simulink model "foc_hfi"  (R2023a)
settings: Solver=FixedStepAuto  StartTime=0.0  StopTime=1  FixedStep=1e-6  MaxStep=0.00001  RelTol=1e-3
undefined symbols (not defined in the file): DiscIntNeverNeededParam
libraries: slpidlib x4, spsAlphaBetaZerotodq0Lib x1, spsDCVoltageSourceLib x1, spsGroundLib x1, dspfdesign x1, spsPermanentMagnetSynchronousMachineLib x1, simulink x1, spsSVPWMGenerator2LevelLib x1, spsUniversalBridgeLib x1, spsabctoAlphaBetaZeroLib x1, spsdq0toAlphaBetaZeroLib x1, sps_lib x1
settings Model: Creator=28076  LastModifiedBy=28076

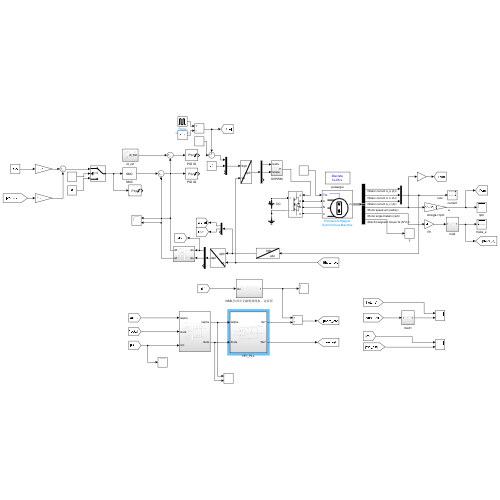
[thumbnail: Simulink's stored preview of the top-level diagram]
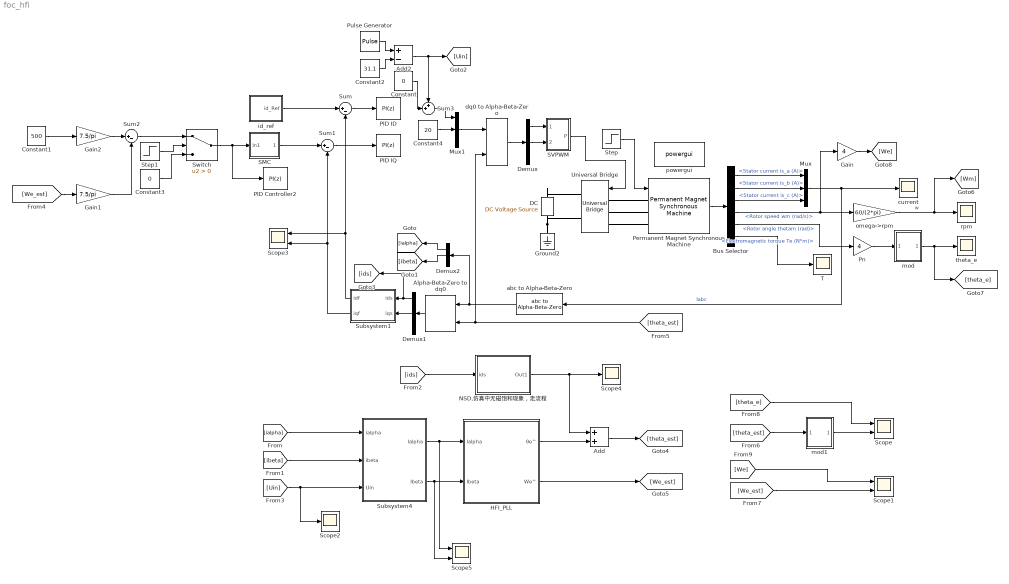
== system foc_hfi ==
  Add : Sum
  Add2 : Sum  Inputs=+-
  Alpha-Beta-Zero to dq0 : spsAlphaBetaZerotodq0Lib/Alpha-Beta-Zero to dq0  Alignment=Aligned with phase A axis
  Bus Selector : BusSelector  OutputSignals=Stator current is_a (A),Stator current is_b (A),Stator current is_c (A),Rotor speed wm (rad/s),Rotor angle thetam (rad),Electromagnetic torque Te (N*m)
  Constant : Constant  Value=0
  Constant1 : Constant  Value=500
  Constant2 : Constant  Value=31.1
  Constant3 : Constant  Value=0
  Constant4 : Constant  Value=20
  "DC " : spsDCVoltageSourceLib/DC Voltage Source  Amplitude=311  Measurements=None
  Demux : Demux  Outputs=3
  Demux1 : Demux  Outputs=3
  Demux2 : Demux  Outputs=3
  Gain : Gain  Gain=4
  Gain1 : Gain  Gain=7.5/pi
  Gain2 : Gain  Gain=7.5/pi
  Ground2 : spsGroundLib/Ground  LConnTagsString=a
  HFI_PLL : Subsystem
  Mux : Mux  Inputs=3
  Mux1 : Mux  Inputs=3
  NSD,仿真中无磁饱和现象，走流程 : Subsystem
  PID Controller2 : slpidlib/PID Controller  Controller=PI  Form=Parallel  TimeDomain=Discrete-time  UseExternalTs=off  SampleTime=1e-4  IntegratorMethod=Forward Euler  FilterMethod=Forward Euler  ControllerParametersSource=internal  P=0.014  I=0.05  UseKiTs=off  D=0  N=100  UseFilter=on  TunerSelectOption=Transfer Function Based (PID Tuner App)  InitialConditionSource=internal  InitialConditionForIntegrator=0  InitialConditionForFilter=0  DifferentiatorICPrevScaledInput=0  ExternalReset=none  TrackingMode=off  Kt=1  LimitOutput=on  SatLimitsSource=internal  UpperSaturationLimit=21  LowerSaturationLimit=-21  LinearizeAsGain=on  AntiWindupMode=none  Kb=1  LimitIntegrator=off  UpperIntegratorSaturationLimit=inf  LowerIntegratorSaturationLimit=-inf  POutMin=[]  POutMax=[]  IOutMin=[]  IOutMax=[]  DOutMin=[]  DOutMax=[]  NOutMin=[]  NOutMax=[]  SumOutMin=[]  SumOutMax=[]  SaturationOutMin=[]  SaturationOutMax=[]  PParamMin=[]  PParamMax=[]  IParamMin=[]  IParamMax=[]  DParamMin=[]  DParamMax=[]  NParamMin=[]  NParamMax=[]  KbParamMin=[]  KbParamMax=[]  KtParamMin=[]  KtParamMax=[]  KbOutMin=[]  KbOutMax=[]  KtOutMin=[]  KtOutMax=[]  IntegratorOutMin=[]  IntegratorOutMax=[]  FilterOutMin=[]  FilterOutMax=[]  SumI1OutMin=[]  SumI1OutMax=[]  SumI2OutMin=[]  SumI2OutMax=[]  SumI3OutMin=[]  SumI3OutMax=[]  SumI4OutMin=[]  SumI4OutMax=[]  SumDOutMin=[]  SumDOutMax=[]  DifferentiatorOutMin=[]  DifferentiatorOutMax=[]  FilterDiffOutCoefMin=[]  FilterDiffOutCoefMax=[]  ReciprocalOutMin=[]  ReciprocalOutMax=[]  SumDenOutMin=[]  SumDenOutMax=[]  SumNumOutMin=[]  SumNumOutMax=[]  DivideOutMin=[]  DivideOutMax=[]  UdiffTsProdOutMin=[]  UdiffTsProdOutMax=[]  NTsProdOutMin=[]  NTsProdOutMax=[]  UintegralTsProdOutMin=[]  UintegralTsProdOutMax=[]  UngainTsProdOutMin=[]  UngainTsProdOutMax=[]  ClampingZeroOutDataTypeStr=Inherit: Inherit via back propagation  ClampingZeroOutMin=[]  ClampingZeroOutMax=[]  FilterDenConstantOutDataTypeStr=Inherit: Inherit via back propagation  FilterDenConstantOutMin=[]  FilterDenConstantOutMax=[]  PCopyOutDataTypeStr=Inherit: Inherit via back propagation  PCopyOutMin=[]  PCopyOutMax=[]  NCopyOutDataTypeStr=Inherit: Inherit via back propagation  NCopyOutMin=[]  NCopyOutMax=[]  IntegratorContinuousStateAttributes=''  IntegratorStateMustResolveToSignalObject=off  IntegratorRTWStateStorageClass=Auto  FilterContinuousStateAttributes=''  FilterStateMustResolveToSignalObject=off  FilterRTWStateStorageClass=Auto  ParallelPVariant=InternalParameters  IdealPVariant=Disabled  IVariant=InternalParameters  DVariant=Disabled  IntegratorVariant=Discrete  SatVariant=Enabled  AWVariant=Passthrough  PCopyVariant=Disabled  TRVariant=Disabled  FdbkBlocksVariant=Forward  IdealPFdbkVariant=Disabled  SatFdbkVariant=Disabled  DerivativeFilterVariant=Disabled  NVariant=Disabled  NCopyVariant=Disabled_SignalSpec  FilterICVariant=Disabled  IntegratorICVariant=InternalICs  ExternalResetVariant=Disabled  TRSumVariant=Passthrough  SumFdbkVariant=Disabled  SumVariant=Sum_PI  TsampFilterVariant=InternalTs  TsampNgainVariant=Passthrough  TsampIntegralVariant=Disabled_SignalSpec  ExternalSaturationOutDataTypeStr=Inherit: Same as second input
  PID ID : slpidlib/PID Controller  Controller=PI  Form=Parallel  TimeDomain=Discrete-time  UseExternalTs=off  SampleTime=1e-4  IntegratorMethod=Forward Euler  FilterMethod=Forward Euler  ControllerParametersSource=internal  P=1100*5.25e-3  I=1100*0.985  UseKiTs=off  D=0  N=100  UseFilter=on  TunerSelectOption=Transfer Function Based (PID Tuner App)  InitialConditionSource=internal  InitialConditionForIntegrator=0  InitialConditionForFilter=0  DifferentiatorICPrevScaledInput=0  ExternalReset=none  TrackingMode=off  Kt=1  LimitOutput=on  SatLimitsSource=internal  UpperSaturationLimit=311/sqrt(3)  LowerSaturationLimit=-311/sqrt(3)  LinearizeAsGain=on  AntiWindupMode=none  Kb=1  LimitIntegrator=off  UpperIntegratorSaturationLimit=inf  LowerIntegratorSaturationLimit=-inf  POutMin=[]  POutMax=[]  IOutMin=[]  IOutMax=[]  DOutMin=[]  DOutMax=[]  NOutMin=[]  NOutMax=[]  SumOutMin=[]  SumOutMax=[]  SaturationOutMin=[]  SaturationOutMax=[]  PParamMin=[]  PParamMax=[]  IParamMin=[]  IParamMax=[]  DParamMin=[]  DParamMax=[]  NParamMin=[]  NParamMax=[]  KbParamMin=[]  KbParamMax=[]  KtParamMin=[]  KtParamMax=[]  KbOutMin=[]  KbOutMax=[]  KtOutMin=[]  KtOutMax=[]  IntegratorOutMin=[]  IntegratorOutMax=[]  FilterOutMin=[]  FilterOutMax=[]  SumI1OutMin=[]  SumI1OutMax=[]  SumI2OutMin=[]  SumI2OutMax=[]  SumI3OutMin=[]  SumI3OutMax=[]  SumI4OutMin=[]  SumI4OutMax=[]  SumDOutMin=[]  SumDOutMax=[]  DifferentiatorOutMin=[]  DifferentiatorOutMax=[]  FilterDiffOutCoefMin=[]  FilterDiffOutCoefMax=[]  ReciprocalOutMin=[]  ReciprocalOutMax=[]  SumDenOutMin=[]  SumDenOutMax=[]  SumNumOutMin=[]  SumNumOutMax=[]  DivideOutMin=[]  DivideOutMax=[]  UdiffTsProdOutMin=[]  UdiffTsProdOutMax=[]  NTsProdOutMin=[]  NTsProdOutMax=[]  UintegralTsProdOutMin=[]  UintegralTsProdOutMax=[]  UngainTsProdOutMin=[]  UngainTsProdOutMax=[]  ClampingZeroOutDataTypeStr=Inherit: Inherit via back propagation  ClampingZeroOutMin=[]  ClampingZeroOutMax=[]  FilterDenConstantOutDataTypeStr=Inherit: Inherit via back propagation  FilterDenConstantOutMin=[]  FilterDenConstantOutMax=[]  PCopyOutDataTypeStr=Inherit: Inherit via back propagation  PCopyOutMin=[]  PCopyOutMax=[]  NCopyOutDataTypeStr=Inherit: Inherit via back propagation  NCopyOutMin=[]  NCopyOutMax=[]  IntegratorContinuousStateAttributes=''  IntegratorStateMustResolveToSignalObject=off  IntegratorRTWStateStorageClass=Auto  FilterContinuousStateAttributes=''  FilterStateMustResolveToSignalObject=off  FilterRTWStateStorageClass=Auto  ParallelPVariant=InternalParameters  IdealPVariant=Disabled  IVariant=InternalParameters  DVariant=Disabled  IntegratorVariant=Discrete  SatVariant=Enabled  AWVariant=Passthrough  PCopyVariant=Disabled  TRVariant=Disabled  FdbkBlocksVariant=Forward  IdealPFdbkVariant=Disabled  SatFdbkVariant=Disabled  DerivativeFilterVariant=Disabled  NVariant=Disabled  NCopyVariant=Disabled_SignalSpec  FilterICVariant=Disabled  IntegratorICVariant=InternalICs  ExternalResetVariant=Disabled  TRSumVariant=Passthrough  SumFdbkVariant=Disabled  SumVariant=Sum_PI  TsampFilterVariant=InternalTs  TsampNgainVariant=Passthrough  TsampIntegralVariant=Disabled_SignalSpec  ExternalSaturationOutDataTypeStr=Inherit: Same as second input
  PID IQ : slpidlib/PID Controller  Controller=PI  Form=Parallel  TimeDomain=Discrete-time  UseExternalTs=off  SampleTime=1e-4  IntegratorMethod=Forward Euler  FilterMethod=Forward Euler  ControllerParametersSource=internal  P=1100*12e-3  I=1100*0.985  UseKiTs=off  D=0  N=100  UseFilter=on  TunerSelectOption=Transfer Function Based (PID Tuner App)  InitialConditionSource=internal  InitialConditionForIntegrator=0  InitialConditionForFilter=0  DifferentiatorICPrevScaledInput=0  ExternalReset=none  TrackingMode=off  Kt=1  LimitOutput=on  SatLimitsSource=internal  UpperSaturationLimit=311/sqrt(3)  LowerSaturationLimit=-311/sqrt(3)  LinearizeAsGain=on  AntiWindupMode=none  Kb=1  LimitIntegrator=off  UpperIntegratorSaturationLimit=inf  LowerIntegratorSaturationLimit=-inf  POutMin=[]  POutMax=[]  IOutMin=[]  IOutMax=[]  DOutMin=[]  DOutMax=[]  NOutMin=[]  NOutMax=[]  SumOutMin=[]  SumOutMax=[]  SaturationOutMin=[]  SaturationOutMax=[]  PParamMin=[]  PParamMax=[]  IParamMin=[]  IParamMax=[]  DParamMin=[]  DParamMax=[]  NParamMin=[]  NParamMax=[]  KbParamMin=[]  KbParamMax=[]  KtParamMin=[]  KtParamMax=[]  KbOutMin=[]  KbOutMax=[]  KtOutMin=[]  KtOutMax=[]  IntegratorOutMin=[]  IntegratorOutMax=[]  FilterOutMin=[]  FilterOutMax=[]  SumI1OutMin=[]  SumI1OutMax=[]  SumI2OutMin=[]  SumI2OutMax=[]  SumI3OutMin=[]  SumI3OutMax=[]  SumI4OutMin=[]  SumI4OutMax=[]  SumDOutMin=[]  SumDOutMax=[]  DifferentiatorOutMin=[]  DifferentiatorOutMax=[]  FilterDiffOutCoefMin=[]  FilterDiffOutCoefMax=[]  ReciprocalOutMin=[]  ReciprocalOutMax=[]  SumDenOutMin=[]  SumDenOutMax=[]  SumNumOutMin=[]  SumNumOutMax=[]  DivideOutMin=[]  DivideOutMax=[]  UdiffTsProdOutMin=[]  UdiffTsProdOutMax=[]  NTsProdOutMin=[]  NTsProdOutMax=[]  UintegralTsProdOutMin=[]  UintegralTsProdOutMax=[]  UngainTsProdOutMin=[]  UngainTsProdOutMax=[]  ClampingZeroOutDataTypeStr=Inherit: Inherit via back propagation  ClampingZeroOutMin=[]  ClampingZeroOutMax=[]  FilterDenConstantOutDataTypeStr=Inherit: Inherit via back propagation  FilterDenConstantOutMin=[]  FilterDenConstantOutMax=[]  PCopyOutDataTypeStr=Inherit: Inherit via back propagation  PCopyOutMin=[]  PCopyOutMax=[]  NCopyOutDataTypeStr=Inherit: Inherit via back propagation  NCopyOutMin=[]  NCopyOutMax=[]  IntegratorContinuousStateAttributes=''  IntegratorStateMustResolveToSignalObject=off  IntegratorRTWStateStorageClass=Auto  FilterContinuousStateAttributes=''  FilterStateMustResolveToSignalObject=off  FilterRTWStateStorageClass=Auto  ParallelPVariant=InternalParameters  IdealPVariant=Disabled  IVariant=InternalParameters  DVariant=Disabled  IntegratorVariant=Discrete  SatVariant=Enabled  AWVariant=Passthrough  PCopyVariant=Disabled  TRVariant=Disabled  FdbkBlocksVariant=Forward  IdealPFdbkVariant=Disabled  SatFdbkVariant=Disabled  DerivativeFilterVariant=Disabled  NVariant=Disabled  NCopyVariant=Disabled_SignalSpec  FilterICVariant=Disabled  IntegratorICVariant=InternalICs  ExternalResetVariant=Disabled  TRSumVariant=Passthrough  SumFdbkVariant=Disabled  SumVariant=Sum_PI  TsampFilterVariant=InternalTs  TsampNgainVariant=Passthrough  TsampIntegralVariant=Disabled_SignalSpec  ExternalSaturationOutDataTypeStr=Inherit: Same as second input
  Permanent Magnet Synchronous Machine : spsPermanentMagnetSynchronousMachineLib/Permanent Magnet Synchronous Machine  NbPhases=3  FluxDistribution=Sinusoidal  RotorType=Salient-pole  MechanicalLoad=Torque Tm  PresetModel=No  ShowDetailedParameters=on  MeasurementBus=off  Resistance=0.985  Inductance=8.5e-3  dqInductances=[5.25e-3,12e-3]  La=0.0085  MachineConstant=Flux linkage established by magnets (V.s)  Flux=0.1827  VoltageCst=132.5525  TorqueCst=1.0962  Flat=120  Mechanical="[ 3e-3, 0,  4 ]"  PolePairs=4  InitialConditions=[0,15, 0,0]  InitialConditions5ph=[0 0 0 0 0 0]  RefAngle=Aligned with phase A axis (original Park)  IterativeDiscreteModel=Trapezoidal non iterative  TsBlock=-1  TsPowergui=0
  Pn : Gain  Gain=4
  Pulse Generator : DiscretePulseGenerator  PulseType=Time based  Amplitude=62.2  Period=2e-4  PulseWidth=50
  SMC : Subsystem  mask{c=30, q=80, Mu=5, Par_Limits=[30 -30], Init=0, Ts=1e-4}
      mask prompts: c "Gain（c）"; q "Giant（q）"; Par_Limits "Output limits: [ Upper   Lower ]"; Init "Output initial value:"; Ts "Sample time："
      mask DialogControl ParameterGroupVar Prompt: 参数
      mask Display: disp('SMC');
  SVPWM : Subsystem
  Scope{,1,3,5} (4 alike) : Scope  NumInputPorts=2
  Scope2 : Scope
  Scope4 : Scope
  Step : Step  Time=0.025  After=0  SampleTime=0
  Step1 : Step  Time=0.2  SampleTime=0
  Subsystem1 : Subsystem
  Subsystem4 : Subsystem
  Sum : Sum  Inputs=|+-
  Sum1 : Sum  Inputs=|+-
  Sum2 : Sum  Inputs=|+-
  Sum3 : Sum  Inputs=++|
  Switch : Switch  Criteria=u2 > Threshold  SaturateOnIntegerOverflow=off  InputSameDT=off
  T : Scope
  Universal Bridge : spsUniversalBridgeLib/Universal Bridge  Arms=3  SnubberResistance=100  SnubberCapacitance=1e-5  Device=MOSFET / Diodes  Ron=1e-3  Lon=0  ForwardVoltages="[  0  0  ]"  ForwardVoltage=0  GTOparameters=[ 10e-6 , 20e-6 ]  IGBTparameters=[ 1e-6 , 2e-6 ]  Measurements=None  Measurements_2=None  converterType=Rectifier
  abc to Alpha-Beta-Zero : spsabctoAlphaBetaZeroLib/abc to Alpha-Beta-Zero
  current : Scope
  dq0 to Alpha-Beta-Zero : spsdq0toAlphaBetaZeroLib/dq0 to Alpha-Beta-Zero  Alignment=Aligned with phase A axis
  id_ref : Subsystem
  mod : Subsystem
  mod1 : Subsystem
  omega->rpm : Gain  Gain=60/(2*pi)
  powergui : sps_lib/powergui  Priority=1  SimulationMode=Discrete  SampleTime=1e-6  frequency=60  Iterations=50  frequencyindice=0  Pbase=100e6  ErrMax=1e-4  UnitsV=kV  UnitsW=MW  buscounter=0  FunctionMessages=off  echomessages=off  EnableUseOfTLC=off  CurrentSourceSwitches=off  DisableSnubberDevices=off  DisableRonSwitches=off  DisableVfSwitches=off  DisplayEquations=off  AutomaticDiscreteSolvers=off  SolverType=Tustin/Backward Euler (TBE)  Interpol=off  ExternalGateDelay=off  methode=off  Ts=100  x0status=blocks  SPID=on  SwTol=0  HookPort=off  NonlinearTolerance=1e-4  nMaxIteration=100  ContinueOnMaxIteration=off  RestoreLinks=warning  ResistiveCurrentMeasurement=off  Frange=[0:2:500]  Ylog=off  Xlog=on  ShowGrid=off  save=off  variable=ZData  structure=0  ZoomFFT=off  StartTime=0.0  cycles=1  DisplayStyle=1  fundamental=60  FreqAxis=off  MaxFrequency=1000  frequencyindicesteady=1  RmsSteady=1  display=off
  rpm : Scope
  theta_e : Scope
  wires:
  Alpha-Beta-Zero to dq0/1 -> Demux1/1
  Bus Selector/4 -> Gain/1, omega->rpm/1  "<Rotor speed wm (rad/s)>"
  Bus Selector/5 -> Pn/1  "<Rotor angle thetam (rad)>"
  Mux/1 -> abc to Alpha-Beta-Zero/1, current/1  "Iabc"
  omega->rpm/1 -> [Wm], rpm/1  "w"
  Mux1/1 -> dq0 to Alpha-Beta-Zero/1
  Gain2/1 -> Sum2/1
  Sum/1 -> PID ID/1
  Step/1 -> Permanent Magnet Synchronous Machine/1
  Bus Selector/2 -> Mux/2  "<Stator current is_b (A)>"
  Bus Selector/6 -> T/1  "<Electromagnetic torque Te (N*m)>"
  Bus Selector/1 -> Mux/1  "<Stator current is_a (A)>"
  mod/1(Out1) -> [theta_e], theta_e/1
  SVPWM/1(P) -> Universal Bridge/1
  Demux/1 -> SVPWM/1(Ualfa)
  Pn/1 -> mod/1(In1)
  Permanent Magnet Synchronous Machine/1 -> Bus Selector/1
  dq0 to Alpha-Beta-Zero/1 -> Demux/1
  Bus Selector/3 -> Mux/3  "<Stator current is_c (A)>"
  Demux/2 -> SVPWM/2(Ubeta)
  abc to Alpha-Beta-Zero/1 -> Demux2/1, Alpha-Beta-Zero to dq0/1
  Demux2/1 -> [ialpha]
  Demux2/2 -> [ibeta]
  Sum1/1 -> PID IQ/1
  [ialpha] -> Subsystem4/1(ialpha)
  [ibeta] -> Subsystem4/2(ibeta)
  [Uin] -> Scope2/1, Subsystem4/3(Uin)
  Demux1/2 -> Subsystem1/2(iqs)
  Demux1/1 -> [ids], Subsystem1/1(ids)
  Subsystem1/1(idf) -> Sum/2, Scope3/1
  Subsystem1/2(iqf) -> Scope3/2, Sum1/2
  [ids] -> NSD,仿真中无磁饱和现象，走流程/1(ids)
  HFI_PLL/2(We^) -> [We_est]
  Add/1 -> [theta_est]
  Constant3/1 -> Switch/3
  Switch/1 -> PID Controller2/1, SMC/1(In1)
  Step1/1 -> Switch/2
  Sum2/1 -> Switch/1
  [theta_est] -> mod1/1(In1)
  [We_est] -> Scope1/2
  Sum3/1 -> Mux1/1
  [theta_e] -> Scope/1
  HFI_PLL/1(θe^) -> Add/2
  [We] -> Scope1/1
  Gain/1 -> [We]
  [We_est] -> Gain1/1
  mod1/1(Out1) -> Scope/2
  NSD,仿真中无磁饱和现象，走流程/1(Out1) -> Scope4/1, Add/1
  [theta_est] -> Alpha-Beta-Zero to dq0/2, dq0 to Alpha-Beta-Zero/2
  Subsystem4/1(Ialpha) -> Scope5/1, HFI_PLL/1(Ialpha)
  Subsystem4/2(Ibeta) -> Scope5/2, HFI_PLL/2(Ibeta)
  Pulse Generator/1 -> Add2/1
  Constant2/1 -> Add2/2
  id_ref/1(id_Ref) -> Sum/1
  Add2/1 -> Sum3/1, [Uin]
  Gain1/1 -> Sum2/2
  Constant1/1 -> Gain2/1
  SMC/1(Out1) -> Sum1/1
  Constant/1 -> Sum3/2
  Constant4/1 -> Mux1/2
  connections:
  Ground2/LConn1 -- "DC "/LConn1 -- Universal Bridge/RConn2
  Permanent Magnet Synchronous Machine/LConn1 -- Universal Bridge/LConn1
  Permanent Magnet Synchronous Machine/LConn3 -- Universal Bridge/LConn3
  "DC "/RConn1 -- Universal Bridge/RConn1
  Permanent Magnet Synchronous Machine/LConn2 -- Universal Bridge/LConn2

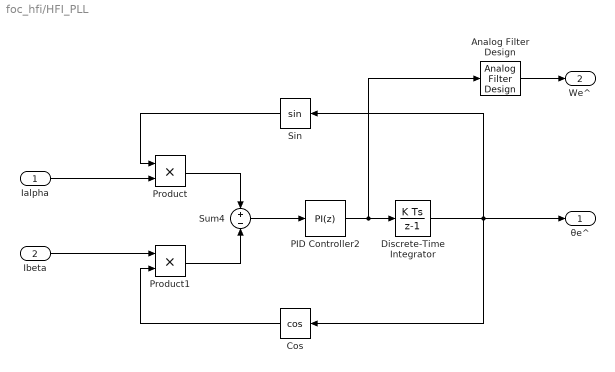
== system foc_hfi/HFI_PLL ==
  Ialpha : Inport
  Ibeta : Inport  Port=2
  Analog Filter Design : dspfdesign/Analog Filter Design  method=Butterworth  filttype=Lowpass  N=3  Wlo=250  Whi=80  Rp=2  Rs=40
  Cos : Trigonometry  Operator=cos
  Discrete-Time Integrator : DiscreteIntegrator  SampleTime=1e-4  ICPrevOutput=DiscIntNeverNeededParam  ICPrevScaledInput=DiscIntNeverNeededParam
  PID Controller2 : slpidlib/PID Controller  Controller=PI  Form=Parallel  TimeDomain=Discrete-time  UseExternalTs=off  SampleTime=1e-4  IntegratorMethod=Forward Euler  FilterMethod=Forward Euler  ControllerParametersSource=internal  P=2200  I=1210000  UseKiTs=off  D=0  N=100  UseFilter=on  TunerSelectOption=Transfer Function Based (PID Tuner App)  InitialConditionSource=internal  InitialConditionForIntegrator=0  InitialConditionForFilter=0  DifferentiatorICPrevScaledInput=0  ExternalReset=none  TrackingMode=off  Kt=1  LimitOutput=off  SatLimitsSource=internal  UpperSaturationLimit=inf  LowerSaturationLimit=-inf  LinearizeAsGain=on  AntiWindupMode=none  Kb=1  LimitIntegrator=off  UpperIntegratorSaturationLimit=inf  LowerIntegratorSaturationLimit=-inf  POutMin=[]  POutMax=[]  IOutMin=[]  IOutMax=[]  DOutMin=[]  DOutMax=[]  NOutMin=[]  NOutMax=[]  SumOutMin=[]  SumOutMax=[]  SaturationOutMin=[]  SaturationOutMax=[]  PParamMin=[]  PParamMax=[]  IParamMin=[]  IParamMax=[]  DParamMin=[]  DParamMax=[]  NParamMin=[]  NParamMax=[]  KbParamMin=[]  KbParamMax=[]  KtParamMin=[]  KtParamMax=[]  KbOutMin=[]  KbOutMax=[]  KtOutMin=[]  KtOutMax=[]  IntegratorOutMin=[]  IntegratorOutMax=[]  FilterOutMin=[]  FilterOutMax=[]  SumI1OutMin=[]  SumI1OutMax=[]  SumI2OutMin=[]  SumI2OutMax=[]  SumI3OutMin=[]  SumI3OutMax=[]  SumI4OutMin=[]  SumI4OutMax=[]  SumDOutMin=[]  SumDOutMax=[]  DifferentiatorOutMin=[]  DifferentiatorOutMax=[]  FilterDiffOutCoefMin=[]  FilterDiffOutCoefMax=[]  ReciprocalOutMin=[]  ReciprocalOutMax=[]  SumDenOutMin=[]  SumDenOutMax=[]  SumNumOutMin=[]  SumNumOutMax=[]  DivideOutMin=[]  DivideOutMax=[]  UdiffTsProdOutMin=[]  UdiffTsProdOutMax=[]  NTsProdOutMin=[]  NTsProdOutMax=[]  UintegralTsProdOutMin=[]  UintegralTsProdOutMax=[]  UngainTsProdOutMin=[]  UngainTsProdOutMax=[]  ClampingZeroOutDataTypeStr=Inherit: Inherit via back propagation  ClampingZeroOutMin=[]  ClampingZeroOutMax=[]  FilterDenConstantOutDataTypeStr=Inherit: Inherit via back propagation  FilterDenConstantOutMin=[]  FilterDenConstantOutMax=[]  PCopyOutDataTypeStr=Inherit: Inherit via back propagation  PCopyOutMin=[]  PCopyOutMax=[]  NCopyOutDataTypeStr=Inherit: Inherit via back propagation  NCopyOutMin=[]  NCopyOutMax=[]  IntegratorContinuousStateAttributes=''  IntegratorStateMustResolveToSignalObject=off  IntegratorRTWStateStorageClass=Auto  FilterContinuousStateAttributes=''  FilterStateMustResolveToSignalObject=off  FilterRTWStateStorageClass=Auto  ParallelPVariant=InternalParameters  IdealPVariant=Disabled  IVariant=InternalParameters  DVariant=Disabled  IntegratorVariant=Discrete  SatVariant=Disabled  AWVariant=Passthrough  PCopyVariant=Disabled  TRVariant=Disabled  FdbkBlocksVariant=Forward  IdealPFdbkVariant=Disabled  SatFdbkVariant=Disabled  DerivativeFilterVariant=Disabled  NVariant=Disabled  NCopyVariant=Disabled_SignalSpec  FilterICVariant=Disabled  IntegratorICVariant=InternalICs  ExternalResetVariant=Disabled  TRSumVariant=Passthrough  SumFdbkVariant=Disabled  SumVariant=Sum_PI  TsampFilterVariant=InternalTs  TsampNgainVariant=Passthrough  TsampIntegralVariant=Disabled_SignalSpec  ExternalSaturationOutDataTypeStr=Inherit: Same as second input
  Product : Product
  Product1 : Product
  Sin : Trigonometry
  Sum4 : Sum  Inputs=+|-
  θe^ : Outport
  We^ : Outport  Port=2
  wires:
  Discrete-Time Integrator/1 -> θe^/1, Sin/1, Cos/1
  Ibeta/1 -> Product1/1
  PID Controller2/1 -> Analog Filter Design/1, Discrete-Time Integrator/1
  Ialpha/1 -> Product/2
  Sum4/1 -> PID Controller2/1
  Cos/1 -> Product1/2
  Sin/1 -> Product/1
  Product/1 -> Sum4/1
  Product1/1 -> Sum4/2
  Analog Filter Design/1 -> We^/1

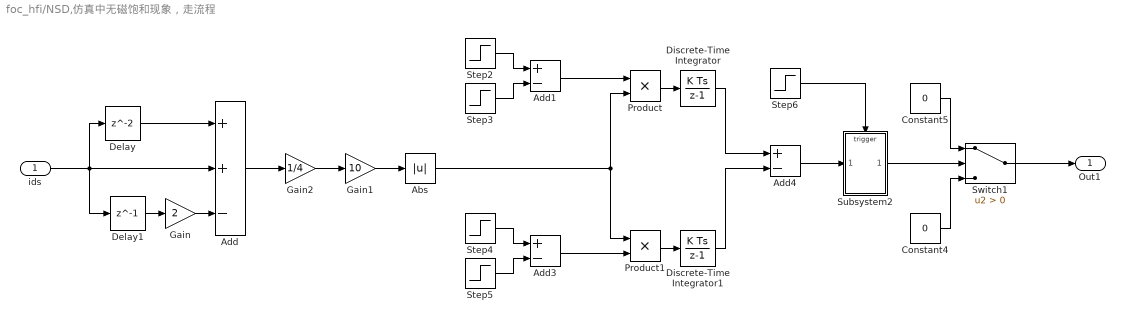
== system foc_hfi/NSD,仿真中无磁饱和现象，走流程 ==
  ids : Inport
  Abs : Abs  SaturateOnIntegerOverflow=off
  Add : Sum  Inputs=++-
  Add1 : Sum  Inputs=+-
  Add3 : Sum  Inputs=+-
  Add4 : Sum  Inputs=+-
  Constant4 : Constant  Value=0
  Constant5 : Constant  Value=0
  Delay : Delay  SampleTime=0.0001
  Delay1 : Delay  DelayLength=1  SampleTime=0.0001
  Discrete-Time Integrator : DiscreteIntegrator  SampleTime=1e-4  ICPrevOutput=DiscIntNeverNeededParam  ICPrevScaledInput=DiscIntNeverNeededParam
  Discrete-Time Integrator1 : DiscreteIntegrator  SampleTime=1e-4  ICPrevOutput=DiscIntNeverNeededParam  ICPrevScaledInput=DiscIntNeverNeededParam
  Gain : Gain  Gain=2
  Gain1 : Gain  Gain=10
  Gain2 : Gain  Gain=1/4
  Product : Product
  Product1 : Product
  Step2 : Step  Time=0.1  SampleTime=0
  Step3 : Step  Time=0.11  SampleTime=0
  Step4 : Step  Time=0.13  SampleTime=0
  Step5 : Step  Time=0.14  SampleTime=0
  Step6 : Step  Time=0.15  SampleTime=0
  Subsystem2 : Subsystem
  Switch1 : Switch  Criteria=u2 > Threshold  SaturateOnIntegerOverflow=off  InputSameDT=off
  Out1 : Outport
  wires:
  Add1/1 -> Product/1
  Step5/1 -> Add3/2
  Subsystem2/1(Out1) -> Switch1/2
  Step4/1 -> Add3/1
  Switch1/1 -> Out1/1
  Step3/1 -> Add1/2
  Product1/1 -> Discrete-Time Integrator1/1
  ids/1 -> Delay/1, Add/2, Delay1/1
  Abs/1 -> Product/2, Product1/1
  Delay1/1 -> Gain/1
  Gain1/1 -> Abs/1
  Add3/1 -> Product1/2
  Constant5/1 -> Switch1/1
  Product/1 -> Discrete-Time Integrator/1
  Gain/1 -> Add/3
  Add4/1 -> Subsystem2/1(In1)
  Delay/1 -> Add/1
  Add/1 -> Gain2/1
  Gain2/1 -> Gain1/1
  Step2/1 -> Add1/1
  Step6/1 -> Subsystem2/Trigger
  Constant4/1 -> Switch1/3
  Discrete-Time Integrator/1 -> Add4/1
  Discrete-Time Integrator1/1 -> Add4/2

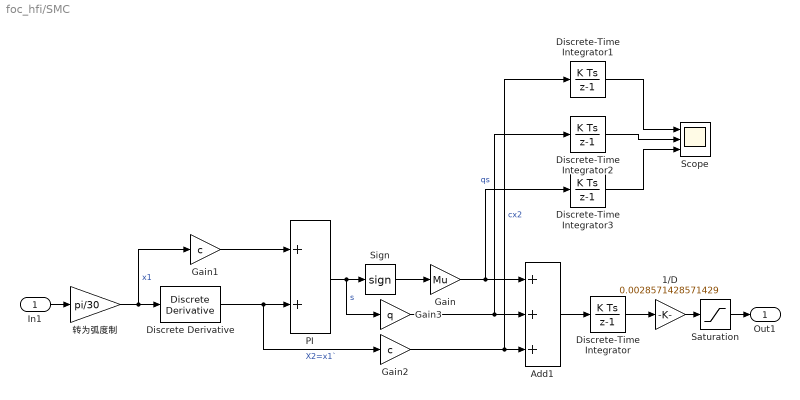
== system foc_hfi/SMC ==
  In1 : Inport
  1/D : Gain  Gain=0.0028571428571429
  Add1 : Sum  Inputs=+++
  Discrete Derivative : simulink/Discrete/Discrete Derivative  gainval=1.0  ICPrevScaledInput=0.0  OutMin=[]  OutMax=[]  OutDataType=fixdt(1, 16)  OutScaling=2^-10  DoSatur=off
  Discrete-Time Integrator{,1..3} (4 alike) : DiscreteIntegrator  SampleTime=1e-4  ICPrevOutput=DiscIntNeverNeededParam  ICPrevScaledInput=DiscIntNeverNeededParam
  Gain : Gain  Gain=Mu
  Gain1 : Gain  Gain=c
  Gain2 : Gain  Gain=c
  Gain3 : Gain  Gain=q
  PI : Sum
  Saturation : Saturate  UpperLimit=30  LowerLimit=-30
  Scope : Scope  NumInputPorts=3
  Sign : Signum
  转为弧度制 : Gain  Gain=pi/30
  Out1 : Outport
  wires:
  PI/1 -> Gain3/1, Sign/1  "s"
  Discrete-Time Integrator/1 -> 1/D/1
  Gain3/1 -> Discrete-Time Integrator2/1, Add1/2  "qs"
  Discrete Derivative/1 -> Gain2/1, PI/2  "X2=x1`"
  Gain/1 -> Discrete-Time Integrator3/1, Add1/1
  转为弧度制/1 -> Gain1/1, Discrete Derivative/1  "x1"
  Add1/1 -> Discrete-Time Integrator/1
  Sign/1 -> Gain/1
  Gain2/1 -> Discrete-Time Integrator1/1, Add1/3  "cx2"
  Gain1/1 -> PI/1
  In1/1 -> 转为弧度制/1
  Discrete-Time Integrator2/1 -> Scope/2
  Discrete-Time Integrator3/1 -> Scope/3
  Discrete-Time Integrator1/1 -> Scope/1
  1/D/1 -> Saturation/1
  Saturation/1 -> Out1/1

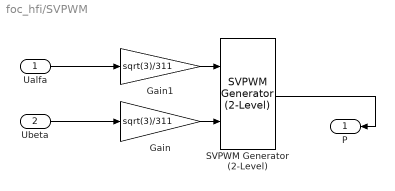
== system foc_hfi/SVPWM ==
  Ualfa : Inport
  Ubeta : Inport  Port=2
  Gain : Gain  Gain=sqrt(3)/311
  Gain1 : Gain  Gain=sqrt(3)/311
  SVPWM Generator (2-Level) : spsSVPWMGenerator2LevelLib/SVPWM Generator (2-Level)  InputType=alpha-beta components  SwitchingPattern=Pattern #1  Fc=10000  ParUref=[0.8 -30 50]  Ts=0
  P : Outport
  wires:
  Gain/1 -> SVPWM Generator (2-Level)/2
  Gain1/1 -> SVPWM Generator (2-Level)/1
  Ubeta/1 -> Gain/1
  SVPWM Generator (2-Level)/1 -> P/1
  Ualfa/1 -> Gain1/1

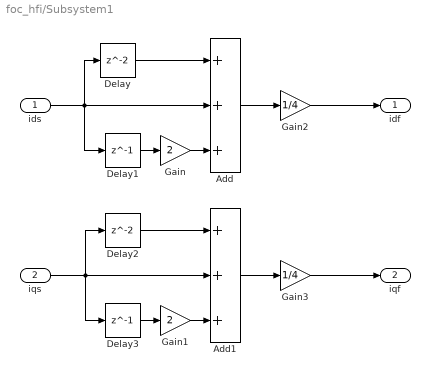
== system foc_hfi/Subsystem1 ==
  ids : Inport
  iqs : Inport  Port=2
  Add : Sum  Inputs=+++
  Add1 : Sum  Inputs=+++
  Delay : Delay  SampleTime=1e-4
  Delay1 : Delay  DelayLength=1  SampleTime=1e-4
  Delay2 : Delay  SampleTime=1e-4
  Delay3 : Delay  DelayLength=1  SampleTime=1e-4
  Gain : Gain  Gain=2
  Gain1 : Gain  Gain=2
  Gain2 : Gain  Gain=1/4
  Gain3 : Gain  Gain=1/4
  idf : Outport
  iqf : Outport  Port=2
  wires:
  Delay3/1 -> Gain1/1
  ids/1 -> Delay/1, Add/2, Delay1/1
  Gain1/1 -> Add1/3
  Delay1/1 -> Gain/1
  Gain/1 -> Add/3
  iqs/1 -> Add1/2, Delay2/1, Delay3/1
  Delay/1 -> Add/1
  Add1/1 -> Gain3/1
  Delay2/1 -> Add1/1
  Add/1 -> Gain2/1
  Gain2/1 -> idf/1
  Gain3/1 -> iqf/1

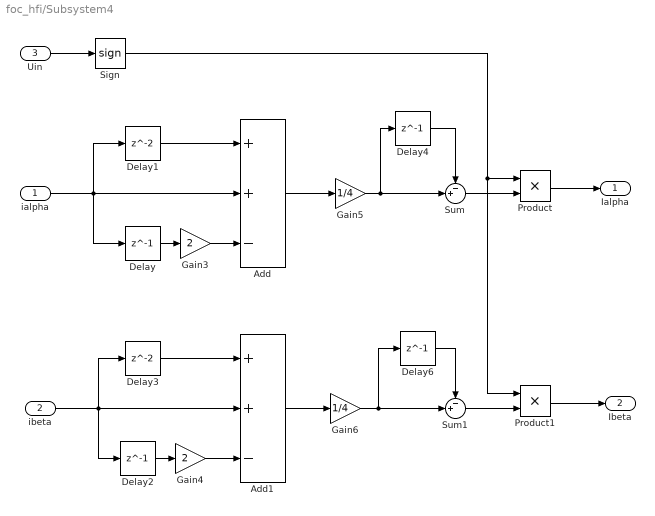
== system foc_hfi/Subsystem4 ==
  ialpha : Inport
  ibeta : Inport  Port=2
  Uin : Inport  Port=3
  Add : Sum  Inputs=++-
  Add1 : Sum  Inputs=++-
  Delay{,2,4,6} (4 alike) : Delay  DelayLength=1  InitialCondition=0  SampleTime=1e-4
  Delay1 : Delay  InitialCondition=0  SampleTime=1e-4
  Delay3 : Delay  InitialCondition=0  SampleTime=1e-4
  Gain3 : Gain  Gain=2
  Gain4 : Gain  Gain=2
  Gain5 : Gain  Gain=1/4
  Gain6 : Gain  Gain=1/4
  Product : Product
  Product1 : Product
  Sign : Signum
  Sum : Sum  Inputs=-+|
  Sum1 : Sum  Inputs=-+|
  Ialpha : Outport
  Ibeta : Outport  Port=2
  wires:
  Product1/1 -> Ibeta/1
  ialpha/1 -> Delay/1, Add/2, Delay1/1
  Gain5/1 -> Delay4/1, Sum/2
  Delay6/1 -> Sum1/1
  Gain6/1 -> Sum1/2, Delay6/1
  Add/1 -> Gain5/1
  Add1/1 -> Gain6/1
  Delay1/1 -> Add/1
  Sum/1 -> Product/2
  Delay3/1 -> Add1/1
  Sum1/1 -> Product1/2
  Delay4/1 -> Sum/1
  Sign/1 -> Product1/1, Product/1
  Uin/1 -> Sign/1
  Product/1 -> Ialpha/1
  ibeta/1 -> Delay2/1, Add1/2, Delay3/1
  Gain4/1 -> Add1/3
  Delay2/1 -> Gain4/1
  Delay/1 -> Gain3/1
  Gain3/1 -> Add/3

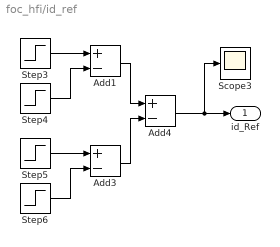
== system foc_hfi/id_ref ==
  Add1 : Sum  Inputs=+-
  Add3 : Sum  Inputs=+-
  Add4 : Sum  Inputs=+-
  Scope3 : Scope
  Step3 : Step  Time=0.1  After=10  SampleTime=0
  Step4 : Step  Time=0.11  After=10  SampleTime=0
  Step5 : Step  Time=0.13  After=10  SampleTime=0
  Step6 : Step  Time=0.14  After=10  SampleTime=0
  id_Ref : Outport
  wires:
  Step3/1 -> Add1/1
  Step4/1 -> Add1/2
  Step5/1 -> Add3/1
  Add1/1 -> Add4/1
  Add4/1 -> Scope3/1, id_Ref/1
  Step6/1 -> Add3/2
  Add3/1 -> Add4/2

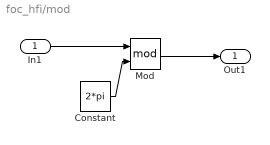
== system foc_hfi/mod ==
  In1 : Inport
  Constant : Constant  Value=2*pi
  Mod : Math  Operator=mod
  Out1 : Outport
  wires:
  Mod/1 -> Out1/1
  Constant/1 -> Mod/2
  In1/1 -> Mod/1

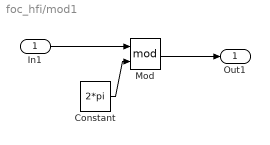
== system foc_hfi/mod1 ==
  In1 : Inport
  Constant : Constant  Value=2*pi
  Mod : Math  Operator=mod
  Out1 : Outport
  wires:
  Mod/1 -> Out1/1
  Constant/1 -> Mod/2
  In1/1 -> Mod/1

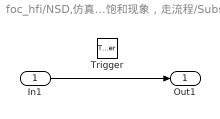
== system foc_hfi/NSD,仿真中无磁饱和现象，走流程/Subsystem2 ==
  In1 : Inport
  Trigger : TriggerPort  VariantControl=(inherit)  PortDimensions=1
  Out1 : Outport
  wires:
  In1/1 -> Out1/1
